simulink model "Pouziti_BUS"  (R2020b)
settings: Solver=VariableStepAuto  StartTime=0.0  StopTime=10.0  RelTol=1e-3  EnableMultiTasking=on
settings Model: Creator=Jirkovsk  LastModifiedBy=jirkovsky
settings DataIOCC: LimitDataPoints=on  SaveFormat=Array  ReturnWorkspaceOutputs=off
settings OptimizationCC: LifeSpan=inf
settings DebuggingCC: UnderspecifiedInitializationDetection=Classic  MergeDetectMultiDrivingBlocksExec=none  SolverPrmCheckMsg=warning  SFUnexpectedBacktrackingDiag=warning  SFNoUnconditionalDefaultTransitionDiag=warning  SFExecutionAtInitializationDiag=none  ArithmeticOperatorsInVariantConditions=warning
settings HardwareCC: ProdBitPerPointer=32  ProdBitPerSizeT=32  ProdBitPerPtrDiffT=32  ProdLargestAtomicFloat=None  ProdIntDivRoundTo=Undefined  ProdEndianess=Unspecified  ProdWordSize=32  ProdHWDeviceType=32-bit Generic
settings ModelReferenceCC: PropagateSignalLabelsOutOfModel=off
settings SFSimCC: SimUseLocalCustomCode=off  CustomCodeUndefinedFunction=UseInterfaceOnly
settings RTWCC: RTWUseLocalCustomCode=off
settings CodeAppCC: StateflowObjectComments=on
settings GRTTargetCC: TargetLangStandard=C89/C90 (ANSI)
settings ConfigComp: CovMetricSettings=dw  CovSaveCumulativeToWorkspaceVar=on  CovSaveSingleToWorkspaceVar=on  CovExternalEMLEnable=off  CovSFcnEnable=off

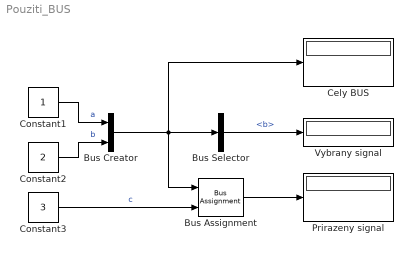
== system Pouziti_BUS ==
  Bus Assignment : BusAssignment  AssignedSignals=b
  Bus Creator : BusCreator  Inputs=2
  Bus Selector : BusSelector  OutputSignals=b
  Cely BUS : Display
  Constant1 : Constant
  Constant2 : Constant  Value=2
  Constant3 : Constant  Value=3
  Prirazeny signal : Display
  Vybrany signal : Display
  wires:
  Constant1/1 -> Bus Creator/1  "a"
  Constant2/1 -> Bus Creator/2  "b"
  Bus Creator/1 -> Cely BUS/1, Bus Assignment/1, Bus Selector/1
  Bus Selector/1 -> Vybrany signal/1  "<b>"
  Constant3/1 -> Bus Assignment/2  "c"
  Bus Assignment/1 -> Prirazeny signal/1
